simulink model "clik2015b"  (R2015b)
settings: Solver=FixedStepDiscrete  StartTime=0.0  StopTime=tfsim  FixedStep=T  RelTol=1e-3
values from neighbouring files (symbols this model uses):
  Kp = diag([500 500 500 50])    [Approccio1.m]    (also in Approccio2.m = 10*diag([50 50 50 5]); Approccio3.m = 10*diag([50 50 50 5]); InversioneCinematica.m = diag([100 100 10 10]); PDpiuGravita.m = 1200*[1;1;1;1;1;1])
  q0 = [0 0 0 0 0 0]'    [Approccio1.m]    (also in Approccio2.m; Approccio3.m; main.m; main2.m)
undefined symbols (not defined in the file or in its folder): cindirSim, DiscIntNeverNeededParam, pinvJ, q0p
settings Model: Creator=Giovanni  LastModifiedBy=Giovanni
settings ConfigComp: CovModelRefEnable=Off

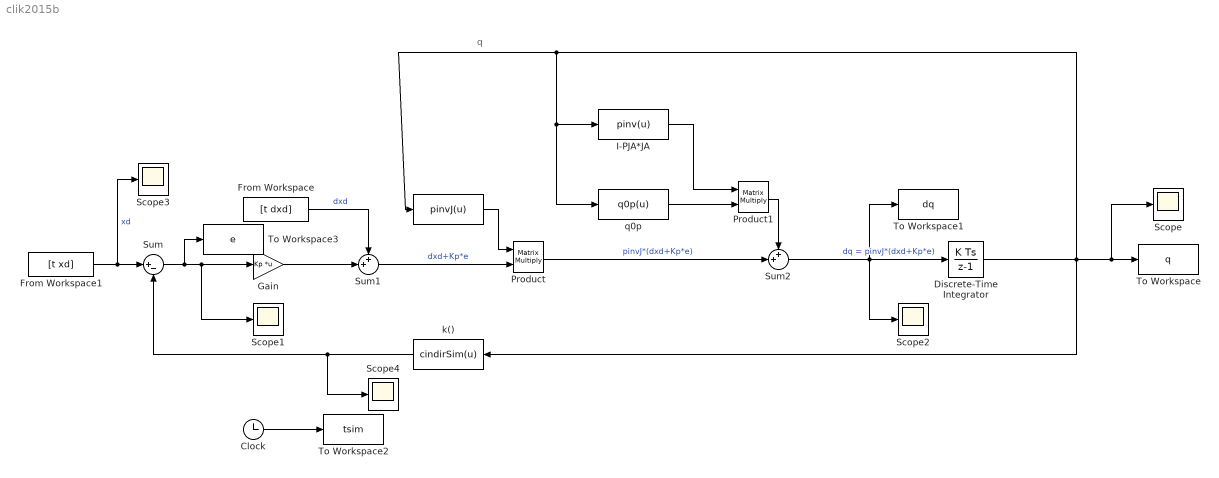
== system clik2015b ==
  note: q
  " " : MATLABFcn  MATLABFcn=pinvJ(u)  OutputDimensions=[6 4]  Output1D=off
      mask Display: disp('pinvJ')
  Clock : Clock
  Discrete-Time Integrator : DiscreteIntegrator  InitialCondition=q0  InitialConditionSetting=State (most efficient)  SampleTime=-1  ICPrevOutput=DiscIntNeverNeededParam  ICPrevScaledInput=DiscIntNeverNeededParam
  From Workspace : FromWorkspace  VariableName=[t dxd]  OutputAfterFinalValue=Setting to zero
  From Workspace1 : FromWorkspace  VariableName=[t xd]  SampleTime=0  OutputAfterFinalValue=Holding final value
  Gain : Gain  Gain=Kp  Multiplication=Matrix(K*u)
  I-PJA*JA : MATLABFcn  MATLABFcn=pinv(u)  OutputDimensions=[6 6]  Output1D=off
      mask Display: disp('P')
  Product : Product  Multiplication=Matrix(*)
  Product1 : Product  Multiplication=Matrix(*)
  Scope{,1..4} (5 alike) : Scope
  Sum : Sum  Inputs=|+-
  Sum1 : Sum  Inputs=++|
  Sum2 : Sum  Inputs=++|
  To Workspace : ToWorkspace  VariableName=q  SampleTime=-1
  To Workspace1 : ToWorkspace  VariableName=dq  SampleTime=-1
  To Workspace2 : ToWorkspace  VariableName=tsim  SampleTime=-1
  To Workspace3 : ToWorkspace  VariableName=e  SampleTime=-1
  k() : MATLABFcn  MATLABFcn=cindirSim(u)  OutputDimensions=[4,1]  Output1D=off
      mask Display: disp('k()')
  q0p : MATLABFcn  MATLABFcn=q0p(u)  OutputDimensions=[6 1]  Output1D=off
      mask Display: disp('q0p')
  wires:
  Sum/1 -> To Workspace3/1, Scope1/1, Gain/1
  Gain/1 -> Sum1/2
  From Workspace1/1 -> Scope3/1, Sum/1  "xd"
  k()/1 -> Scope4/1, Sum/2
  From Workspace/1 -> Sum1/1  "dxd"
  Sum1/1 -> Product/2  "dxd+Kp*e"
  Sum2/1 -> Scope2/1, To Workspace1/1, Discrete-Time Integrator/1  "dq = pinvJ*(dxd+Kp*e)"
  " "/1 -> Product/1
  Clock/1 -> To Workspace2/1
  Product/1 -> Sum2/2  "pinvJ*(dxd+Kp*e)"
  Discrete-Time Integrator/1 -> q0p/1, I-PJA*JA/1, " "/1, Scope/1, To Workspace/1, k()/1
  I-PJA*JA/1 -> Product1/1
  Product1/1 -> Sum2/1
  q0p/1 -> Product1/2
